simulink library "NPC_lib"  (R2023b)
settings: Solver=VariableStepAuto  StartTime=0.0  StopTime=10.0  RelTol=1e-3
settings Model: Creator=timsp  LastModifiedBy=timsp

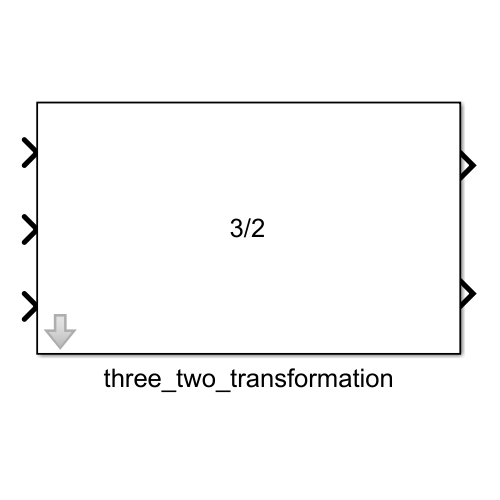
[thumbnail: Simulink's stored preview of the top-level diagram]
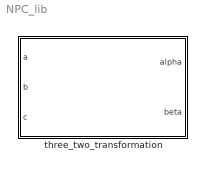
== system NPC_lib ==
  three_two_transformation : Subsystem
      mask Help: 3 / 2 Transformation für Raumzeigerdarstellung
      mask Display: disp('3/2');

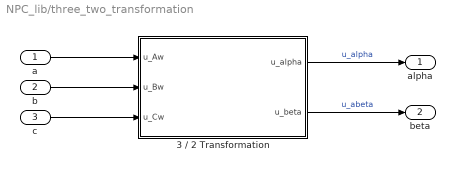
== system NPC_lib/three_two_transformation ==
  a : Inport
  b : Inport  Port=2
  c : Inport  Port=3
  3 / 2 Transformation : MATLAB Function  TreatAsAtomicUnit=on
  alpha : Outport
  beta : Outport  Port=2
  wires:
  c/1 -> 3 / 2 Transformation/3(u_Cw)
  3 / 2 Transformation/1(u_alpha) -> alpha/1  "u_alpha"
  b/1 -> 3 / 2 Transformation/2(u_Bw)
  3 / 2 Transformation/2(u_beta) -> beta/1  "u_abeta"
  a/1 -> 3 / 2 Transformation/1(u_Aw)

== matlab function NPC_lib/three_two_transformation/3 // 2 Transformation ==
  data: u_Aw input; u_alpha output; u_Bw input; u_Cw input; u_beta output
function [u_alpha, u_beta] = fcn(u_Aw, u_Bw, u_Cw)
% ### input vector ###
% u1 = u_Aw
% u2 = u_Bw
% u3 = u_Cw

% ### output vector ###
% y1 = u_alpha
% y2 = u_beta
% y3 = u_0

% ### calculation ###
    T = 2/3.*   [1 -1/2 -1/2;...
                0 sqrt(3)/2 -sqrt(3)/2;...
                1/2 1/2 1/2];
    
    y = T * [u_Aw; u_Bw; u_Cw];   
% ### return ###
    u_alpha = y(1);
    u_beta = y(2);
    %u_0 = y(3);
end
